simulink model "Uebung10_2_v2016a"  (R2016a)
settings: Solver=VariableStepAuto  SolverMode=SingleTasking  StartTime=0.0  StopTime=10000000  RelTol=1e-3
undefined symbols (not defined in the file or in its folder): entity, getCurrSimTime, showValue
settings Model: Creator=gome  LastModifiedBy=gome
settings DebuggingCC: SFUnexpectedBacktrackingDiag=error  SFNoUnconditionalDefaultTransitionDiag=error
settings GRTTargetCC: TargetLangStandard=C99 (ISO)  GeneratePreprocessorConditionals=Use local settings
settings ConfigComp: CovMetricSettings=dwe  CovHtmlReporting=off  CovSaveCumulativeToWorkspaceVar=off  CovSaveSingleToWorkspaceVar=off  CovExternalEMLEnable=on

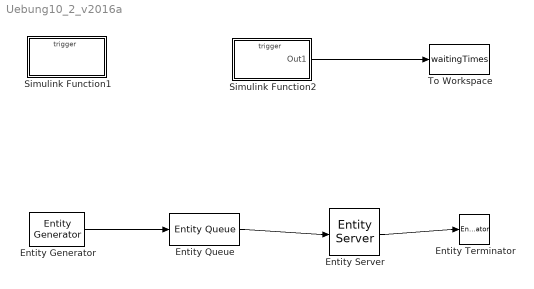
== system Uebung10_2_v2016a ==
  Entity Generator : EntityGenerator  OutputPortMessageModes=m  TimeSource=MATLAB action  IntergenerationTimeAction=|  GenerateAction=entity.startTime = getCurrSimTime;  AttributeName=startTime  EntityType=Structured  EntityTypeName=Entity
      | persistent init
      | if isempty(init)
      |     init = 1;
      |     rng(1);
      | end
      | 
      | dt = exprnd(1/30*3600);
  Entity Queue : EntityQueue  InputPortMessageModes=m  OutputPortMessageModes=m  Capacity=inf
      settings: OutputPortMap=o5
  Entity Server : EntityServer  InputPortMessageModes=m  OutputPortMessageModes=m  Capacity=6  ServiceTimeSource=MATLAB action  ServiceTimeAction=|  EntryAction=showValue(getCurrSimTime-entity.startTime);
      | persistent init
      | if isempty(init)
      |     init = 1;
      |     rng(09593);
      | end
      | 
      | dt = exprnd(5*60);
  Entity Terminator : EntityTerminator  InputPortMessageModes=m
  Simulink Function1 : Subsystem  TreatAsAtomicUnit=on
  Simulink Function2 : Subsystem  TreatAsAtomicUnit=on
  To Workspace : ToWorkspace  VariableName=waitingTimes  SampleTime=-1
  wires:
  Entity Queue/1 -> Entity Server/1
  Entity Generator/1 -> Entity Queue/1
  Entity Server/1 -> Entity Terminator/1
  Simulink Function2/1(Out1) -> To Workspace/1

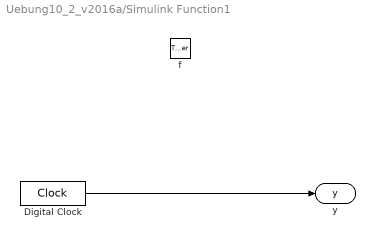
== system Uebung10_2_v2016a/Simulink Function1 ==
  f : TriggerPort  TriggerType=function-call  IsSimulinkFunction=on  FunctionName=getCurrSimTime  VariantControl=Variant
  Digital Clock : DigitalClock  SampleTime=-1
  y : ArgOut  DisableCoverage=on  ArgumentName=y
  wires:
  Digital Clock/1 -> y/1

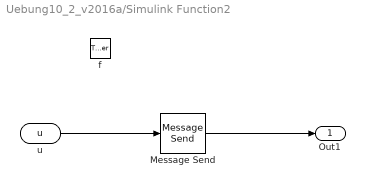
== system Uebung10_2_v2016a/Simulink Function2 ==
  f : TriggerPort  TriggerType=function-call  IsSimulinkFunction=on  FunctionName=showValue  VariantControl=Variant
  Message Send : MessageSend  OutputPortMessageModes=m
      settings: InputPortMap=u1
  u : ArgIn  DisableCoverage=on  ArgumentName=u
  Out1 : Outport
  wires:
  u/1 -> Message Send/1
  Message Send/1 -> Out1/1
